simulink model "innoPWM_TestBench"  (R2022a)
settings: Solver=VariableStepAuto  StartTime=0.0  StopTime=0.5  FixedStep=1e-10  MaxStep=1e-4  RelTol=1e-3
PreLoadFcn:
  | clear;
  | dead_time= 5e-7;
  | T_sample = 1e-7;
  | fpwm= 8e3;
  | fel=200;
  | amplitude=0.1;
  | U_dc=800;
  | Iq_soll=200;
  | 
  | load('busdef.mat')
  | 
  | %**** Controller ****
  | L_filter = 70e-6;
  | R_losses = 1.74e-3;
  | PGain = L_filter*0.05*2*pi;
  | IGain = R_losses*0.05*2*pi;
  | 
  | %**** Deadtime Correction ****
  | Rds_on_module = 0.045/15;
  | 
  | %**** Filter ****
  | FilterQuality = 0.7071
InitFcn:
  | %%PGain = (L_filter*0.09*2*pi*f_pwm-R_losses)*0.45;
  | %%IGain = PGain*50/1.2; %% 25 = Period for ringing with too hight PGain
  | 
  | %%PGain = L_filter/(2*(1.5/fpwm));
  | %%IGain  = PGain*R_losses/L_filter;
undefined symbols (not defined in the file): DiscIntNeverNeededParam
libraries: nesl_utility x12, simulink x10, fl_lib x7, ee_lib x7, eeTransforms x2, spsFirstOrderFilterLib x1, spsRMSLib x1, simulink_extras x1, spspowerguiLib x1
settings Model: VariantFading=off  Creator=Z634594  LastModifiedBy=z634594
settings SolverCC: ZeroCrossAlgorithm=Adaptive  AlgebraicLoopSolver=TrustRegion
settings DataIOCC: ReturnWorkspaceOutputs=off
settings DebuggingCC: MergeDetectMultiDrivingBlocksExec=none  UnconnectedInputMsg=warning  UnconnectedOutputMsg=warning  UnconnectedLineMsg=warning  SFMachineParentedDataDiag=warning  ArithmeticOperatorsInVariantConditions=warning
settings SFSimCC: SimUseLocalCustomCode=off  CustomCodeUndefinedFunction=UseInterfaceOnly
settings RTWCC: RTWUseLocalCustomCode=off  DLArmComputeVersion=19.05
settings CodeAppCC: StateflowObjectComments=on

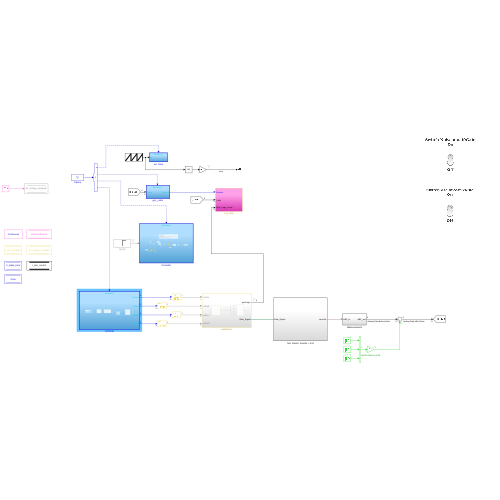
[thumbnail: Simulink's stored preview of the top-level diagram]
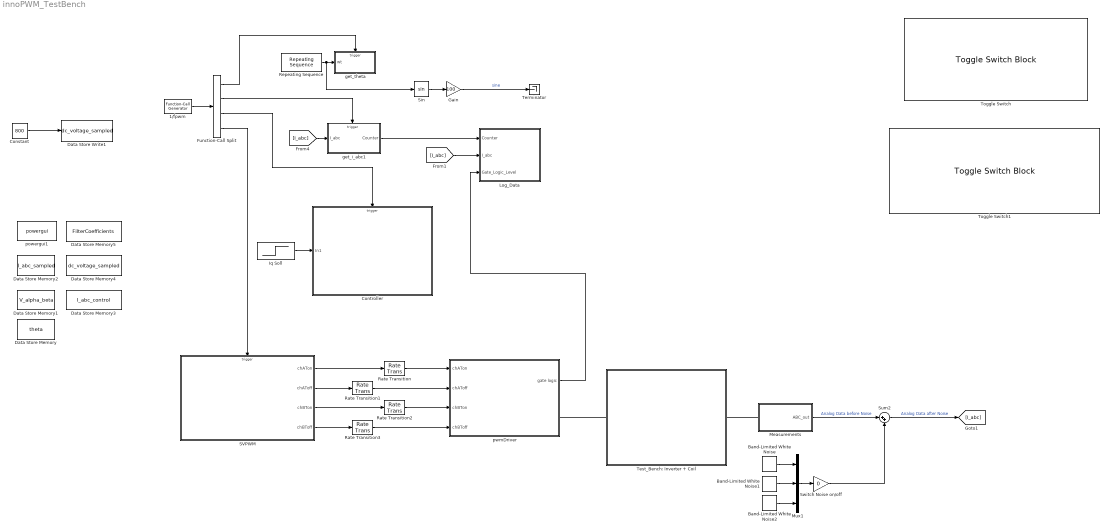
== system innoPWM_TestBench ==
  1/fpwm : simulink/Ports & Subsystems/Function-Call Generator  sample_time=1/fpwm  numberOfIterations=1  DisallowWideOutput=off
  Band-Limited White Noise : simulink/Sources/Band-Limited White Noise  Cov=[0.0004]  Ts=pi/2*1e-6  seed=[40000]
  Band-Limited White Noise1 : simulink/Sources/Band-Limited White Noise  Cov=[0.0004]  Ts=pi/2*1e-6  seed=[35000]
  Band-Limited White Noise2 : simulink/Sources/Band-Limited White Noise  Cov=[0.0004]  Ts=pi/2*1e-6  seed=[30000]
  Constant : Constant  Value=800
  Controller : Subsystem  TreatAsAtomicUnit=on
  Data Store Memory : DataStoreMemory  DataStoreName=theta  ReadBeforeWriteMsg=warning  WriteAfterWriteMsg=warning  WriteAfterReadMsg=warning  ShowAdditionalParam=off
  Data Store Memory1 : DataStoreMemory  DataStoreName=V_alpha_beta  ReadBeforeWriteMsg=warning  WriteAfterWriteMsg=warning  WriteAfterReadMsg=warning  InitialValue=[0 0]  ShowAdditionalParam=off
  Data Store Memory2 : DataStoreMemory  DataStoreName=I_abc_sampled  ReadBeforeWriteMsg=warning  WriteAfterWriteMsg=warning  WriteAfterReadMsg=warning  InitialValue=[0 0 0]  ShowAdditionalParam=off
  Data Store Memory3 : DataStoreMemory  DataStoreName=I_abc_control  ReadBeforeWriteMsg=warning  WriteAfterWriteMsg=warning  WriteAfterReadMsg=warning  InitialValue=[0 0 0]  ShowAdditionalParam=off
  Data Store Memory4 : DataStoreMemory  DataStoreName=dc_voltage_sampled  ReadBeforeWriteMsg=warning  WriteAfterWriteMsg=warning  WriteAfterReadMsg=warning  InitialValue=U_dc  ShowAdditionalParam=off
  Data Store Memory5 : DataStoreMemory  DataStoreName=FilterCoefficients  ReadBeforeWriteMsg=warning  WriteAfterWriteMsg=warning  WriteAfterReadMsg=warning  InitialValue=[1 0 0 0 0]  ShowAdditionalParam=off
  Data Store Write1 : DataStoreWrite  DataStoreName=dc_voltage_sampled  IndexOptions=Index vector (dialog)  Indices=1  OutputSizes=1
  Function-Call Split : FunctionCallSplit  IconShape=distinctive  NumOutputPorts=4  OutputPortLayout=default
  Gain : Gain  Gain=100
  Iq Soll : Step  Time=0.001  After=70  SampleTime=0
  Log_Data : Subsystem
  Measurements : Subsystem
  Mux1 : Mux  Inputs=3
  Rate Transition{,1..3} (4 alike) : RateTransition
  Repeating Sequence : simulink/Sources/Repeating Sequence  rep_seq_t=[0 1/fel]  rep_seq_y=[0 2*pi]
  SVPWM : Subsystem
  Sin : Trigonometry
  Sum2 : Sum  Inputs=|++
  Switch Noise on/off : Gain  Gain=0
  Terminator : Terminator
  Test_Bench: Inverter + Coil : Subsystem
  Toggle Switch : ToggleSwitchBlock
      settings: Values={{'Off', 'On'}, [0 1]}
  Toggle Switch1 : ToggleSwitchBlock
      settings: Values={{'Off', 'On'}, [0 1]}
  get_i_abc1 : Subsystem  TreatAsAtomicUnit=on
  get_theta : Subsystem  TreatAsAtomicUnit=on
  powergui1 : spspowerguiLib/powergui  Priority=1  SimulationMode=Continuous  SampleTime=1e-9  frequency=60  Iterations=50  frequencyindice=0  Pbase=100e6  ErrMax=1e-4  UnitsV=kV  UnitsW=MW  buscounter=0  FunctionMessages=off  echomessages=off  EnableUseOfTLC=off  CurrentSourceSwitches=off  DisableSnubberDevices=off  DisableRonSwitches=off  DisableVfSwitches=off  DisplayEquations=off  AutomaticDiscreteSolvers=off  SolverType=Tustin/Backward Euler (TBE)  Interpol=off  ExternalGateDelay=off  methode=off  Ts=100  x0status=blocks  SPID=on  SwTol=0  HookPort=off  NonlinearTolerance=1e-4  nMaxIteration=100  ContinueOnMaxIteration=off  RestoreLinks=warning  ResistiveCurrentMeasurement=off  Frange=[0:2:500]  Ylog=off  Xlog=on  ShowGrid=off  save=off  variable=ZData  structure=logsout  ZoomFFT=off  StartTime=0.01  cycles=10  DisplayStyle=1  fundamental=200  FreqAxis=off  MaxFrequency=10000  frequencyindicesteady=1  RmsSteady=1  display=off
  pwmDriver : Subsystem
  wires:
  Repeating Sequence/1 -> Sin/1, get_theta/1(wt)
  [I_abc] -> Log_Data/2(I_abc)
  Sum2/1 -> [I_abc]  "Analog Data after Noise"
  Band-Limited White Noise1/1 -> Mux1/2
  Band-Limited White Noise/1 -> Mux1/1
  Band-Limited White Noise2/1 -> Mux1/3
  Mux1/1 -> Switch Noise on/off/1
  Measurements/1(ABC_out) -> Sum2/1  "Analog Data before Noise"
  Switch Noise on/off/1 -> Sum2/2
  Constant/1 -> Data Store Write1/1
  get_i_abc1/1(Counter) -> Log_Data/1(Counter)
  pwmDriver/1(gate logic) -> Log_Data/3(Gate_Logic_Level)
  [I_abc] -> get_i_abc1/1(I_abc)
  1/fpwm/1 -> Function-Call Split/1
  Function-Call Split/1 -> get_theta/Trigger
  Function-Call Split/2 -> get_i_abc1/Trigger
  Function-Call Split/3 -> Controller/Trigger
  Function-Call Split/4 -> SVPWM/Trigger
  SVPWM/4(chBToff) -> Rate Transition3/1
  SVPWM/3(chBTon) -> Rate Transition2/1
  SVPWM/2(chAToff) -> Rate Transition1/1
  SVPWM/1(chATon) -> Rate Transition/1
  Rate Transition/1 -> pwmDriver/1(chATon)
  Rate Transition1/1 -> pwmDriver/2(chAToff)
  Rate Transition2/1 -> pwmDriver/3(chBTon)
  Rate Transition3/1 -> pwmDriver/4(chBToff)
  Sin/1 -> Gain/1
  Gain/1 -> Terminator/1  "sine"
  Iq Soll/1 -> Controller/1(In1)
  connections:
  Test_Bench: Inverter + Coil/LConn1 -- pwmDriver/RConn1
  Measurements/LConn1 -- Test_Bench: Inverter + Coil/RConn1

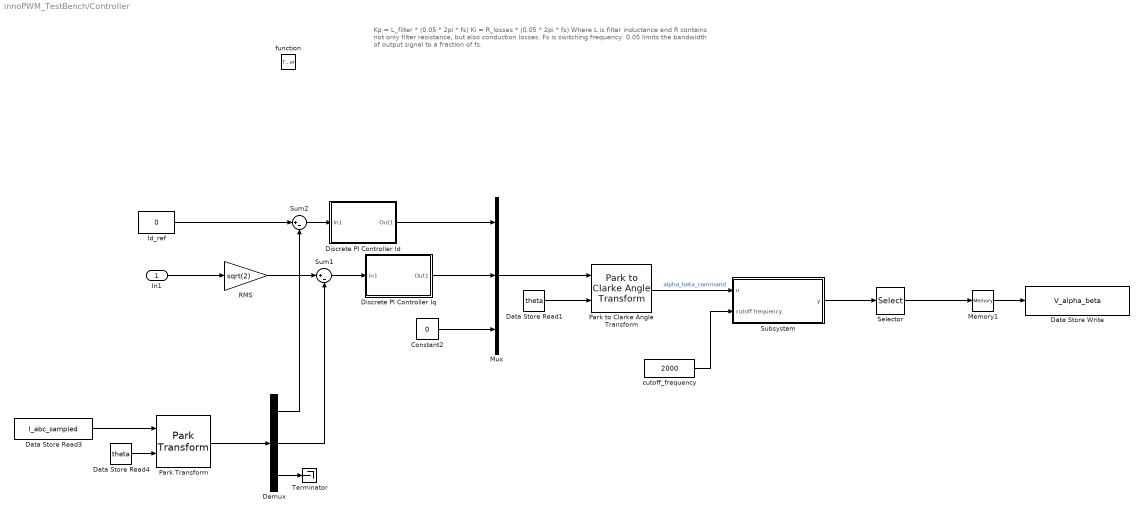
== system innoPWM_TestBench/Controller ==
  note: Kp = L_filter * (0.05 * 2pi * fs)
      |
      | Ki = R_losses * (0.05 * 2pi * fs)
      |
      | Where L is filter inductance and R contains not only filter resistance, but also conduction losses.
      | Fs is switching frequency.
      | 0.05 limits the bandwidth of output signal to a fraction of fs.
  In1 : Inport
  function : TriggerPort  TriggerType=function-call  VariantControl=Variant
  Constant2 : Constant  Value=0
  Data Store Read1 : DataStoreRead  DataStoreName=theta  IndexOptions=Index vector (dialog)  Indices=1  OutputSizes=1
  Data Store Read3 : DataStoreRead  DataStoreName=I_abc_sampled  IndexOptions=Index vector (dialog)  Indices=1  OutputSizes=1
  Data Store Read4 : DataStoreRead  DataStoreName=theta  IndexOptions=Index vector (dialog)  Indices=1  OutputSizes=1
  Data Store Write : DataStoreWrite  DataStoreName=V_alpha_beta  IndexOptions=Index vector (dialog)  Indices=1  OutputSizes=1
  Demux : Demux  Outputs=3
  Discrete PI Controller Id : Subsystem
  Discrete PI Controller Iq : Subsystem
  Id_ref : Constant  Value=0
  Memory1 : Memory  InheritSampleTime=on  LinearizeAsDelay=on
  Mux : Mux  Inputs=3
  Park Transform : eeTransforms/Park Transform  AxisAlignment=Q-axis  PowerInvariant=off
  Park to Clarke Angle Transform : eeTransforms/Park to Clarke Angle Transform  AxisAlignment=Q-axis
      settings: SourceProductBaseCode=PS
  RMS : Gain  Gain=sqrt(2)
  Selector : Selector  InputPortWidth=3  IndexOptions=Index vector (dialog)  Indices=[1 2]  OutputSizes=1
  Subsystem : Subsystem
  Sum1 : Sum  Inputs=|+-
  Sum2 : Sum  Inputs=|+-
  Terminator : Terminator
  cutoff_frequency : Constant  Value=2000
  wires:
  Demux/1 -> Sum2/2
  Mux/1 -> Park to Clarke Angle Transform/1
  Demux/3 -> Terminator/1
  Demux/2 -> Sum1/2
  Constant2/1 -> Mux/3
  Sum2/1 -> Discrete PI Controller Id/1(In1)
  Sum1/1 -> Discrete PI Controller Iq/1(In1)
  Discrete PI Controller Iq/1(Out1) -> Mux/2
  Data Store Read3/1 -> Park Transform/1
  Data Store Read4/1 -> Park Transform/2
  Data Store Read1/1 -> Park to Clarke Angle Transform/2
  Memory1/1 -> Data Store Write/1
  Discrete PI Controller Id/1(Out1) -> Mux/1
  Park Transform/1 -> Demux/1
  Selector/1 -> Memory1/1
  Id_ref/1 -> Sum2/1
  In1/1 -> RMS/1
  RMS/1 -> Sum1/1
  cutoff_frequency/1 -> Subsystem/2(cutoff frequency)
  Park to Clarke Angle Transform/1 -> Subsystem/1(u)  "alpha_beta_command"
  Subsystem/1(y) -> Selector/1

== system innoPWM_TestBench/Log_Data ==
  Counter : Inport
  I_abc : Inport  Port=2
  Gate_Logic_Level : Inport  Port=3
  Data Store Read1 : DataStoreRead  DataStoreName=I_abc_sampled  IndexOptions=Index vector (dialog)  Indices=1  OutputSizes=1
  Data Store Read2 : DataStoreRead  DataStoreName=I_abc_control  IndexOptions=Index vector (dialog)  Indices=1  OutputSizes=1
  Delay : Delay  DelayLength=1  SampleTime=T_sample
  Gain : Gain  Gain=50
  Logical Operator : Logic  Operator=XOR  AllPortsSameDT=off  OutDataTypeStr=boolean
  Product : Product
  Scope1 : Scope  NumInputPorts=3
  Scope6 : Scope  NumInputPorts=5
  wires:
  Delay/1 -> Scope1/2, Logical Operator/1
  Data Store Read1/1 -> Product/2, Scope6/1
  Counter/1 -> Scope1/1, Logical Operator/2, Delay/1
  Product/1 -> Scope6/3
  Logical Operator/1 -> Scope1/3, Product/1
  Gain/1 -> Scope6/4
  I_abc/1 -> Scope6/2
  Gate_Logic_Level/1 -> Gain/1
  Data Store Read2/1 -> Scope6/5

== system innoPWM_TestBench/Measurements ==
  First-Order Filter : spsFirstOrderFilterLib/First-Order Filter  FilterType=Lowpass  Tc=25e-6  Ts=0  Initialize=off  Vac_Init=[0, 0, 60]  Vdc_Init=0  PlotResponse=off  FreqRange="[0,  200,  1]"
  PS-Simulink Converter1 : nesl_utility/PS-Simulink Converter  PhysicalDomain=network_engine_domain  SubClassName=ps_output  LeftPortType=input  RightPortType=output  PseudoPeriodic=off  Frequencies=[]  VectorFormat=1-D array  Unit=1  AffineConversion=off
      settings: SourceProductBaseCode=SS,PW,VE
  RMS : spsRMSLib/RMS  TrueRMS=on  Freq=fel  RMSInit=0  Ts=0
  Terminator : Terminator
  Terminator1 : Terminator
  ABC_in : PMIOPort  Side=Left
  ABC_out : Outport  VectorParamsAs1DForOutWhenUnconnected=off
  wires:
  PS-Simulink Converter1/1 -> RMS/1, First-Order Filter/1, ABC_out/1
  RMS/1 -> Terminator/1  "rmsCurrent3Phase"
  First-Order Filter/1 -> Terminator1/1  "phaseCurrent3Phase"
  connections:
  PS-Simulink Converter1/LConn1 -- ABC_in/RConn1

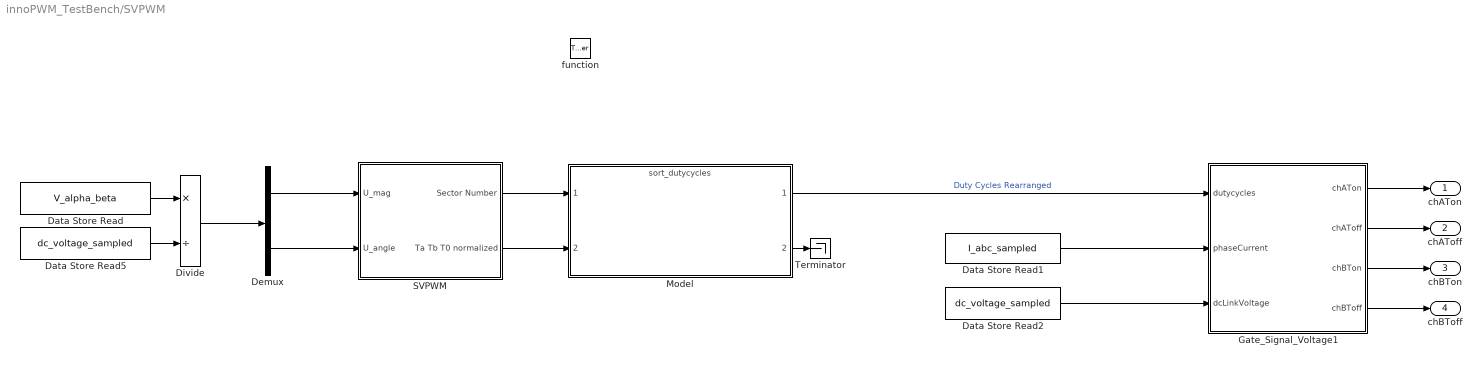
== system innoPWM_TestBench/SVPWM ==
  function : TriggerPort  TriggerType=function-call  VariantControl=(inherit)
  Data Store Read : DataStoreRead  DataStoreName=V_alpha_beta  IndexOptions=Index vector (dialog)  Indices=1  OutputSizes=1
  Data Store Read1 : DataStoreRead  DataStoreName=I_abc_sampled  IndexOptions=Index vector (dialog)  Indices=1  OutputSizes=1
  Data Store Read2 : DataStoreRead  DataStoreName=dc_voltage_sampled  IndexOptions=Index vector (dialog)  Indices=1  OutputSizes=1
  Data Store Read5 : DataStoreRead  DataStoreName=dc_voltage_sampled  IndexOptions=Index vector (dialog)  Indices=1  OutputSizes=1
  Demux : Demux  Outputs=2
  Divide : Product  Inputs=*/
  Gate_Signal_Voltage1 : Subsystem
  Model : ModelReference  ModelNameDialog=sort_dutycycles.slx  SimulationMode=Normal  ModelReferenceVersion=1.5
  SVPWM : Subsystem
  Terminator : Terminator
  chATon : Outport
  chAToff : Outport  Port=2
  chBTon : Outport  Port=3
  chBToff : Outport  Port=4
  wires:
  Divide/1 -> Demux/1
  Data Store Read5/1 -> Divide/2
  SVPWM/1(Sector Number) -> Model/1
  SVPWM/2(Ta Tb T0 normalized) -> Model/2
  Data Store Read/1 -> Divide/1
  Demux/2 -> SVPWM/2(U_angle)
  Model/2 -> Terminator/1
  Demux/1 -> SVPWM/1(U_mag)
  Model/1 -> Gate_Signal_Voltage1/1(dutycycles)  "Duty Cycles Rearranged"
  Data Store Read1/1 -> Gate_Signal_Voltage1/2(phaseCurrent)
  Data Store Read2/1 -> Gate_Signal_Voltage1/3(dcLinkVoltage)
  Gate_Signal_Voltage1/1(chATon) -> chATon/1
  Gate_Signal_Voltage1/2(chAToff) -> chAToff/1
  Gate_Signal_Voltage1/3(chBTon) -> chBTon/1
  Gate_Signal_Voltage1/4(chBToff) -> chBToff/1

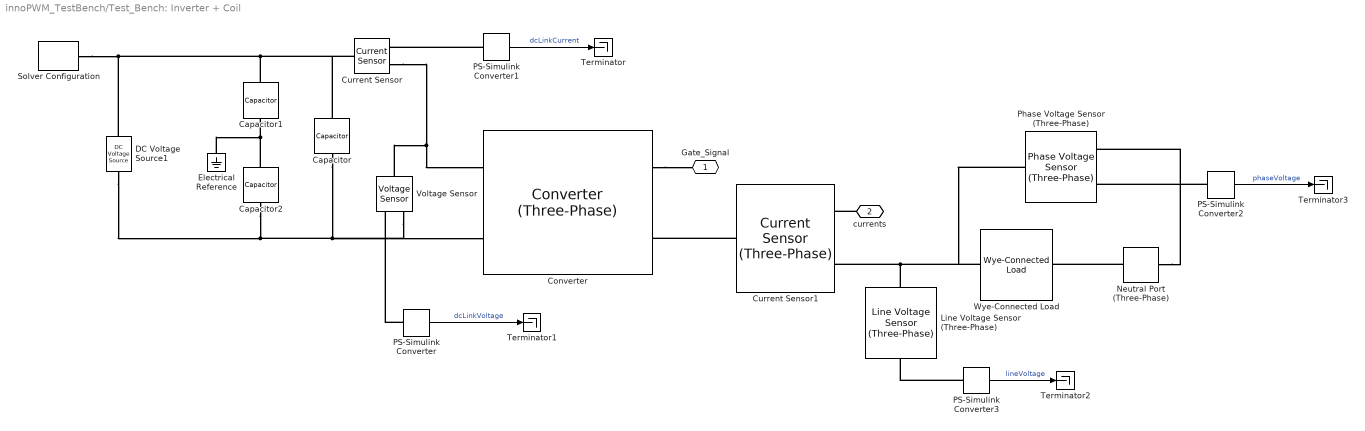
== system innoPWM_TestBench/Test_Bench: Inverter + Coil ==
  Capacitor : fl_lib/Electrical/Electrical Elements/Capacitor  c=550e-6 F  r=1e-6 Ohm  g=0 1/Ohm  i_specify=off  i_priority=None  i=0 A  i_nominal_specify=off  i_nominal_unit=A  i_nominal_value=1  v_specify=off  v_priority=None  v=0 V  v_nominal_specify=off  v_nominal_unit=V  v_nominal_value=1  vc_specify=on  vc_priority=High  vc=U_dc V  vc_nominal_specify=off  vc_nominal_unit=V  vc_nominal_value=1
      settings: SourceProductBaseCode=PW,SS,VE
  Capacitor1 : fl_lib/Electrical/Electrical Elements/Capacitor  c=100e-9 F  r=1e-6 Ohm  g=0 1/Ohm  i_specify=off  i_priority=None  i=0 A  i_nominal_specify=off  i_nominal_unit=A  i_nominal_value=1  v_specify=off  v_priority=None  v=0 V  v_nominal_specify=off  v_nominal_unit=V  v_nominal_value=1  vc_specify=on  vc_priority=High  vc=U_dc/2 V  vc_nominal_specify=off  vc_nominal_unit=V  vc_nominal_value=1
      settings: SourceProductBaseCode=PW,SS,VE
  Capacitor2 : fl_lib/Electrical/Electrical Elements/Capacitor  c=100e-9 F  r=1e-6 Ohm  g=0 1/Ohm  i_specify=off  i_priority=None  i=0 A  i_nominal_specify=off  i_nominal_unit=A  i_nominal_value=1  v_specify=off  v_priority=None  v=0 V  v_nominal_specify=off  v_nominal_unit=V  v_nominal_value=1  vc_specify=on  vc_priority=High  vc=U_dc/2 V  vc_nominal_specify=off  vc_nominal_unit=V  vc_nominal_value=1
      settings: SourceProductBaseCode=PW,SS,VE
  Converter : ee_lib/Semiconductors & Converters/Converters/Converter (Three-Phase)  port_option=ee.enum.threePhasePort.composite  device_type=ee.enum.converters.switchingdevice.mosfet  Vf=0.8 V  Ron=0.001 Ohm  Rds=Rds_on_module Ohm  Goff=1e-9 1/Ohm  Vgt=1 V  Vgt_off=-1 V  Ih=1 A  Vth=4 V  diode_param=ee.enum.converters.protectiondiode.nodynamics  diode_Vf=2 V  diode_Ron=Rds_on_module Ohm  diode_Goff=1e-9 1/Ohm  diode_C=50 nF  diode_iRM=-235 A  diode_iF=300 A  diode_idot=-50 A/us  diode_trr_param=ee.enum.converters.diodetrr.trr_factor  diode_trr_factor=3  diode_trr=15 us  diode_Qrr=1.5e+3 s*uA  snubber_type=ee.enum.converters.snubber.exclude  Cs=1e-6 F  Rs=0.01 Ohm
      settings: SourceProductBaseCode=PS
  Current Sensor : fl_lib/Electrical/Electrical Sensors/Current Sensor
      settings: SourceProductBaseCode=PW,SS,VE
  Current Sensor1 : ee_lib/Sensors & Transducers/Current Sensor (Three-Phase)
  DC Voltage Source1 : fl_lib/Electrical/Electrical Sources/DC Voltage Source  v0=U_dc V
      settings: SourceProductBaseCode=PW,SS,VE
  Electrical Reference : fl_lib/Electrical/Electrical Elements/Electrical Reference
      settings: SourceProductBaseCode=PW,SS,VE
  Line Voltage Sensor (Three-Phase) : ee_lib/Sensors & Transducers/Line Voltage Sensor (Three-Phase)
      settings: SourceProductBaseCode=PS
  Neutral Port (Three-Phase) : ee_lib/Connectors & References/Neutral Port (Three-Phase)  G_parasitic=1e-12 1/Ohm
      settings: SourceProductBaseCode=PS  InternalSimscapePortConfiguration="{\"Bottom\":[],\"Left\":[{\"id\":\"N\",\"label\":\"~\",\"type\":\"foundation.electrical.three_phase\"}],\"Right\":[{\"id\":\"n\",\"label\":\"n\",\"type\":\"foundation.electrical.electrical\"}],\"Top\":[]}"
  PS-Simulink Converter{,1..3} (4 alike) : nesl_utility/PS-Simulink Converter  PhysicalDomain=network_engine_domain  SubClassName=ps_output  LeftPortType=input  RightPortType=output  PseudoPeriodic=off  Frequencies=[]  VectorFormat=1-D array  Unit=1  AffineConversion=off
      settings: SourceProductBaseCode=SS,PW,VE
  Phase Voltage Sensor (Three-Phase) : ee_lib/Sensors & Transducers/Phase Voltage Sensor (Three-Phase)
      settings: SourceProductBaseCode=PS
  Solver Configuration : nesl_utility/Solver Configuration  PhysicalDomain=network_engine_domain  SubClassName=solver  LeftPortType=input  RightPortType=generic  Tones=[]  Harmonics=[]  SimulateNoise=off  Profile=off  UseLocalSampling=off  EnableSwitchedLinearOptims=on  FrequencyDomain=off  UseCCode=off  RelTol=0.001  AbsTol=1e-06  MinStep=1e-09  ToWorkspace=off  RevertToSquareIcSolve=off  NumHomotopyIterations=100  PhasorMode=off  PhasorModeNumHarmonics=1  IndexReductionMethod=DerivativeReplacement  DoDC=off  ResidualTolerance=1e-09  UseLocalSolver=off  LocalSolverChoice=NE_BACKWARD_EULER_ADVANCER  LocalSolverSampleTime=0.001  DoFixedCost=off  MaxNonlinIter=3  MaxModeIter=2  ComputeImpulses=off  ImpulseIterations=2  LinearAlgebra=Sparse  LinearAlgebraNumThread=0  EquationFormulation=NE_TIME_EF  DelaysMemoryBudget=1024  AutomaticFiltering=on  FilteringTimeConstant=0.001  PartitionStorageMethod=AS_NEEDED  PartitionMemoryBudget=1024  PartitionMethod=FAST
      settings: SourceProductBaseCode=SS,PW,VE
  Terminator{,1..3} (4 alike) : Terminator
  Voltage Sensor : fl_lib/Electrical/Electrical Sensors/Voltage Sensor
      settings: SourceProductBaseCode=PW,SS,VE
  Wye-Connected Load : ee_lib/Passive/RLC Assemblies/Wye-Connected Load  parameterization=ee.enum.rlc.parameterization.direct  component_structure=ee.enum.rlc.structure.SeriesRL  component_structure_PQ=ee.enum.rlc.structure.SeriesRL  R=1.74e-3 Ohm  L=70e-6 H  C=1e-6 F  VRated=24e3 V  FRated=60 Hz  P=1e3 W  Qpos=1e2 V*A  Qneg=-1e2 V*A  R_parasitic=1e-6 Ohm  G_parasitic=1e-9 1/Ohm  R_parasitic_PQ=1e-6 Ohm  G_parasitic_PQ=1e-6 1/Ohm  Vmag0=24e3 V  Vang0=0 deg  Freq0=60 Hz  IL_specify=off  IL_priority=High  IL=[ 0 0 0 ] A  IL_nominal_specify=off  IL_nominal_unit=A  IL_nominal_value=1  VC_specify=off  VC_priority=High  VC=[ 0 0 0 ] V  VC_nominal_specify=off  VC_nominal_unit=V  VC_nominal_value=1
      settings: SourceProductBaseCode=PS
  Gate_Signal : PMIOPort  Side=Left
  currents : PMIOPort  Port=2  Side=Right
  wires:
  PS-Simulink Converter1/1 -> Terminator/1  "dcLinkCurrent"
  PS-Simulink Converter/1 -> Terminator1/1  "dcLinkVoltage"
  PS-Simulink Converter3/1 -> Terminator2/1  "lineVoltage"
  PS-Simulink Converter2/1 -> Terminator3/1  "phaseVoltage"
  connections:
  Current Sensor1/LConn1 -- Converter/LConn2
  Converter/LConn1 -- Gate_Signal/RConn1
  Capacitor/RConn1 -- Converter/RConn2 -- Voltage Sensor/RConn2 -- DC Voltage Source1/RConn1 -- Capacitor2/RConn1
  Current Sensor/RConn2 -- Converter/RConn1 -- Voltage Sensor/LConn1
  PS-Simulink Converter/LConn1 -- Voltage Sensor/RConn1
  PS-Simulink Converter1/LConn1 -- Current Sensor/RConn1
  Capacitor1/LConn1 -- Capacitor/LConn1 -- Current Sensor/LConn1 -- DC Voltage Source1/LConn1 -- Solver Configuration/RConn1
  currents/RConn1 -- Current Sensor1/RConn1
  PS-Simulink Converter2/LConn1 -- Phase Voltage Sensor (Three-Phase)/RConn1
  Capacitor2/LConn1 -- Electrical Reference/LConn1 -- Capacitor1/RConn1
  PS-Simulink Converter3/LConn1 -- Line Voltage Sensor (Three-Phase)/RConn1
  Line Voltage Sensor (Three-Phase)/LConn1 -- Wye-Connected Load/LConn1 -- Phase Voltage Sensor (Three-Phase)/LConn1 -- Current Sensor1/RConn2
  Neutral Port (Three-Phase)/LConn1 -- Phase Voltage Sensor (Three-Phase)/RConn2
  Neutral Port (Three-Phase)/RConn1 -- Wye-Connected Load/RConn1

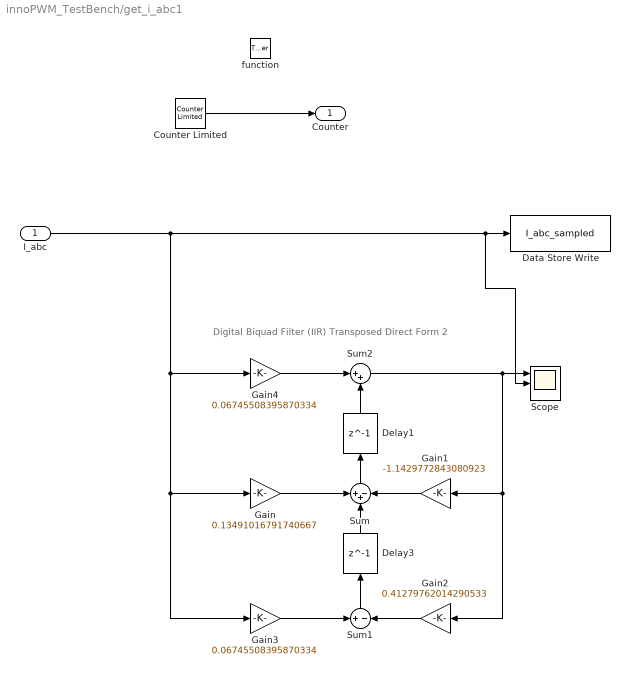
== system innoPWM_TestBench/get_i_abc1 ==
  note: Digital Biquad Filter (IIR)
      | Transposed Direct Form 2
  I_abc : Inport
  function : TriggerPort  TriggerType=function-call  VariantControl=Variant
  Counter Limited : simulink/Sources/Counter Limited  uplimit=1  tsamp=-1
  Data Store Write : DataStoreWrite  DataStoreName=I_abc_sampled  IndexOptions=Index vector (dialog)  Indices=1  OutputSizes=1
  Delay1 : Delay  DelayLength=1
  Delay3 : Delay  DelayLength=1
  Gain : Gain  Gain=0.13491016791740667
  Gain1 : Gain  Gain=-1.1429772843080923
  Gain2 : Gain  Gain=0.41279762014290533
  Gain3 : Gain  Gain=0.06745508395870334
  Gain4 : Gain  Gain=0.06745508395870334
  Scope : Scope  NumInputPorts=3
  Sum : Sum  Inputs=++-
  Sum1 : Sum  Inputs=+|-
  Sum2 : Sum  Inputs=|++
  Counter : Outport  VectorParamsAs1DForOutWhenUnconnected=off
  wires:
  Counter Limited/1 -> Counter/1
  Gain/1 -> Sum/1
  Gain1/1 -> Sum/3
  Gain3/1 -> Sum1/1
  Gain2/1 -> Sum1/2
  Gain4/1 -> Sum2/1
  Delay1/1 -> Sum2/2
  Sum/1 -> Delay1/1
  Delay3/1 -> Sum/2
  Sum1/1 -> Delay3/1
  Sum2/1 -> Gain2/1, Gain1/1, Scope/1
  I_abc/1 -> Scope/2, Data Store Write/1, Gain4/1, Gain/1, Gain3/1

== system innoPWM_TestBench/get_theta ==
  wt : Inport
  function : TriggerPort  TriggerType=function-call  VariantControl=Variant
  Data Store Write : DataStoreWrite  DataStoreName=theta  IndexOptions=Index vector (dialog)  Indices=1  OutputSizes=1
  wires:
  wt/1 -> Data Store Write/1

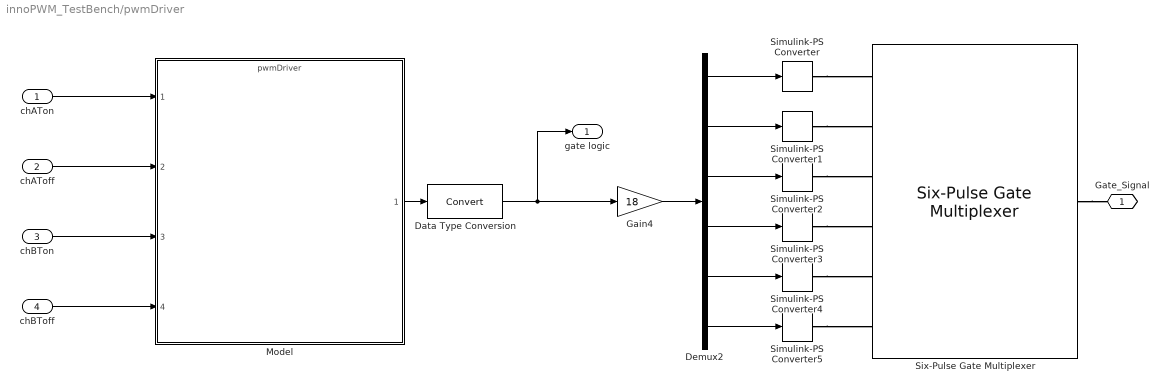
== system innoPWM_TestBench/pwmDriver ==
  chATon : Inport
  chAToff : Inport  Port=2
  chBTon : Inport  Port=3
  chBToff : Inport  Port=4
  Data Type Conversion : DataTypeConversion  SaturateOnIntegerOverflow=off  RndMeth=Floor
  Demux2 : Demux  Outputs=6
  Gain4 : Gain  Gain=18
  Model : ModelReference  ModelNameDialog=pwmDriver.slx  SimulationMode=Normal  ModelReferenceVersion=1.3
  Simulink-PS Converter{,1..5} (6 alike) : nesl_utility/Simulink-PS Converter  PhysicalDomain=network_engine_domain  SubClassName=ps_input  LeftPortType=input  RightPortType=output  PseudoPeriodic=off  Frequencies=[]  NoiseDistribution=none  NoiseParameters=[]  Unit=1  AffineConversion=off  FilteringAndDerivatives=provide  SimscapeFilterOrder=1  InputFilterTimeConstant=0.001  UdotUserProvided=0
      settings: SourceProductBaseCode=SS,PW,VE
  Six-Pulse Gate Multiplexer : ee_lib/Semiconductors & Converters/Converters/Six-Pulse Gate Multiplexer  port_option=ee.enum.controlport.ps
      settings: SourceProductBaseCode=PS
  Gate_Signal : PMIOPort  Side=Right
  gate logic : Outport  VectorParamsAs1DForOutWhenUnconnected=off
  wires:
  chBToff/1 -> Model/4
  Data Type Conversion/1 -> gate logic/1, Gain4/1
  chAToff/1 -> Model/2
  Model/1 -> Data Type Conversion/1
  chBTon/1 -> Model/3
  Gain4/1 -> Demux2/1
  chATon/1 -> Model/1
  Demux2/1 -> Simulink-PS Converter/1
  Demux2/2 -> Simulink-PS Converter1/1
  Demux2/3 -> Simulink-PS Converter2/1
  Demux2/4 -> Simulink-PS Converter3/1
  Demux2/5 -> Simulink-PS Converter4/1
  Demux2/6 -> Simulink-PS Converter5/1
  connections:
  Simulink-PS Converter1/RConn1 -- Six-Pulse Gate Multiplexer/LConn2
  Simulink-PS Converter5/RConn1 -- Six-Pulse Gate Multiplexer/LConn6
  Simulink-PS Converter2/RConn1 -- Six-Pulse Gate Multiplexer/LConn3
  Six-Pulse Gate Multiplexer/RConn1 -- Gate_Signal/RConn1
  Simulink-PS Converter4/RConn1 -- Six-Pulse Gate Multiplexer/LConn5
  Simulink-PS Converter/RConn1 -- Six-Pulse Gate Multiplexer/LConn1
  Simulink-PS Converter3/RConn1 -- Six-Pulse Gate Multiplexer/LConn4

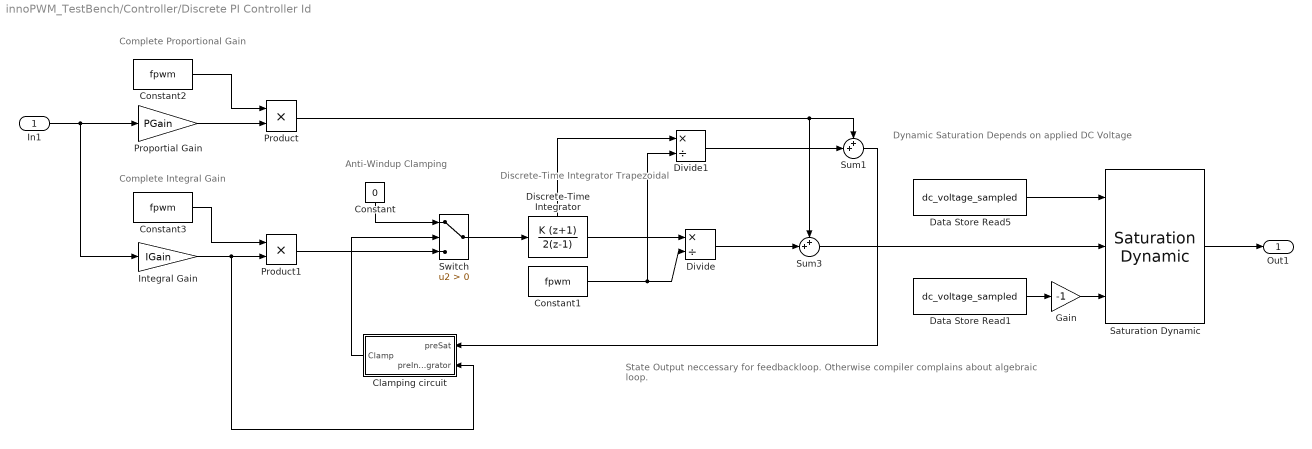
== system innoPWM_TestBench/Controller/Discrete PI Controller Id ==
  note: State Output neccessary for feedbackloop. Otherwise compiler complains about algebraic loop.
  note: Complete Proportional Gain
  note: Discrete-Time Integrator Trapezoidal
  note: Complete Integral Gain
  note: Anti-Windup Clamping
  note: Dynamic Saturation
      | Depends on applied DC Voltage
  In1 : Inport
  Clamping circuit : Subsystem
  Constant : Constant  DisableCoverage=on  Value=0  OutDataTypeStr=Inherit: Inherit via back propagation  PreserveConstantTs=on
  Constant1 : Constant  Value=fpwm
  Constant2 : Constant  Value=fpwm
  Constant3 : Constant  Value=fpwm
  Data Store Read1 : DataStoreRead  DataStoreName=dc_voltage_sampled  IndexOptions=Index vector (dialog)  Indices=1  OutputSizes=1
  Data Store Read5 : DataStoreRead  DataStoreName=dc_voltage_sampled  IndexOptions=Index vector (dialog)  Indices=1  OutputSizes=1
  Discrete-Time Integrator : DiscreteIntegrator  IntegratorMethod=Accumulation: Trapezoidal  SampleTime=-1  ShowStatePort=on  ICPrevOutput=DiscIntNeverNeededParam  ICPrevScaledInput=DiscIntNeverNeededParam
  Divide : Product  Inputs=*/
  Divide1 : Product  Inputs=*/
  Gain : Gain  Gain=-1
  Integral Gain : Gain  Gain=IGain
  Product : Product
  Product1 : Product
  Proportial Gain : Gain  Gain=PGain
  Saturation Dynamic : simulink/Discontinuities/Saturation Dynamic  OutMin=[]  OutMax=[]  OutDataTypeStr=Inherit: Same as second input  OutDataType=fixdt(1, 16)  OutScaling=2^-10  DoSatur=off
  Sum1 : Sum  Inputs=++|
  Sum3 : Sum  Inputs=++|
  Switch : Switch  Criteria=u2 > Threshold  SaturateOnIntegerOverflow=off
  Out1 : Outport  VectorParamsAs1DForOutWhenUnconnected=off
  wires:
  Constant/1 -> Switch/1
  Clamping circuit/1(Clamp) -> Switch/2
  In1/1 -> Proportial Gain/1, Integral Gain/1
  Discrete-Time Integrator/1 -> Divide/1
  Switch/1 -> Discrete-Time Integrator/1
  Constant1/1 -> Divide/2, Divide1/2
  Sum1/1 -> Clamping circuit/1(preSat)
  Data Store Read5/1 -> Saturation Dynamic/1
  Data Store Read1/1 -> Gain/1
  Gain/1 -> Saturation Dynamic/3
  Saturation Dynamic/1 -> Out1/1
  Sum3/1 -> Saturation Dynamic/2
  Proportial Gain/1 -> Product/2
  Constant2/1 -> Product/1
  Integral Gain/1 -> Clamping circuit/2(preIntegrator), Product1/2
  Constant3/1 -> Product1/1
  Divide/1 -> Sum3/2
  Divide1/1 -> Sum1/2
  Discrete-Time Integrator/State -> Divide1/1
  Product/1 -> Sum3/1, Sum1/1
  Product1/1 -> Switch/3

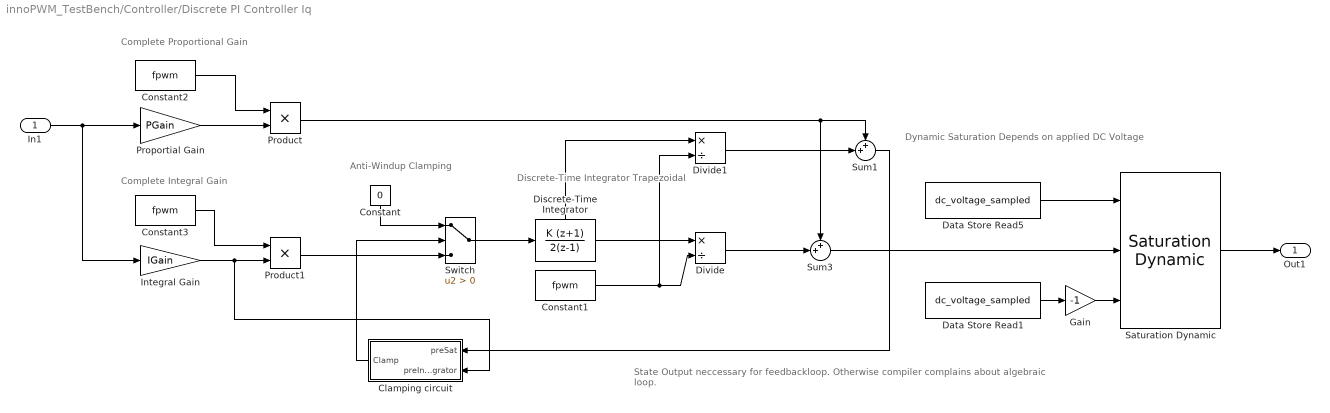
== system innoPWM_TestBench/Controller/Discrete PI Controller Iq ==
  note: Dynamic Saturation
      | Depends on applied DC Voltage
  note: Anti-Windup Clamping
  note: Complete Integral Gain
  note: Discrete-Time Integrator Trapezoidal
  note: Complete Proportional Gain
  note: State Output neccessary for feedbackloop. Otherwise compiler complains about algebraic loop.
  In1 : Inport
  Clamping circuit : Subsystem
  Constant : Constant  DisableCoverage=on  Value=0  OutDataTypeStr=Inherit: Inherit via back propagation  PreserveConstantTs=on
  Constant1 : Constant  Value=fpwm
  Constant2 : Constant  Value=fpwm
  Constant3 : Constant  Value=fpwm
  Data Store Read1 : DataStoreRead  DataStoreName=dc_voltage_sampled  IndexOptions=Index vector (dialog)  Indices=1  OutputSizes=1
  Data Store Read5 : DataStoreRead  DataStoreName=dc_voltage_sampled  IndexOptions=Index vector (dialog)  Indices=1  OutputSizes=1
  Discrete-Time Integrator : DiscreteIntegrator  IntegratorMethod=Accumulation: Trapezoidal  SampleTime=-1  ShowStatePort=on  ICPrevOutput=DiscIntNeverNeededParam  ICPrevScaledInput=DiscIntNeverNeededParam
  Divide : Product  Inputs=*/
  Divide1 : Product  Inputs=*/
  Gain : Gain  Gain=-1
  Integral Gain : Gain  Gain=IGain
  Product : Product
  Product1 : Product
  Proportial Gain : Gain  Gain=PGain
  Saturation Dynamic : simulink/Discontinuities/Saturation Dynamic  OutMin=[]  OutMax=[]  OutDataTypeStr=Inherit: Same as second input  OutDataType=fixdt(1, 16)  OutScaling=2^-10  DoSatur=off
  Sum1 : Sum  Inputs=++|
  Sum3 : Sum  Inputs=++|
  Switch : Switch  Criteria=u2 > Threshold  SaturateOnIntegerOverflow=off
  Out1 : Outport  VectorParamsAs1DForOutWhenUnconnected=off
  wires:
  Constant3/1 -> Product1/1
  Integral Gain/1 -> Clamping circuit/2(preIntegrator), Product1/2
  Constant2/1 -> Product/1
  Proportial Gain/1 -> Product/2
  Saturation Dynamic/1 -> Out1/1
  Gain/1 -> Saturation Dynamic/3
  Data Store Read1/1 -> Gain/1
  Data Store Read5/1 -> Saturation Dynamic/1
  Sum1/1 -> Clamping circuit/1(preSat)
  Constant1/1 -> Divide1/2, Divide/2
  Switch/1 -> Discrete-Time Integrator/1
  Discrete-Time Integrator/1 -> Divide/1
  In1/1 -> Integral Gain/1, Proportial Gain/1
  Clamping circuit/1(Clamp) -> Switch/2
  Constant/1 -> Switch/1
  Divide/1 -> Sum3/2
  Discrete-Time Integrator/State -> Divide1/1
  Divide1/1 -> Sum1/2
  Sum3/1 -> Saturation Dynamic/2
  Product/1 -> Sum3/1, Sum1/1
  Product1/1 -> Switch/3

== system innoPWM_TestBench/Controller/Subsystem ==
  u : Inport
  cutoff frequency : Inport  Port=2
  Constant : Constant  Value=fpwm
  MATLAB Function1 : MATLAB Function  TreatAsAtomicUnit=on
  MATLAB Function2 : MATLAB Function  TreatAsAtomicUnit=on
  Product1 : Product
  Product4 : Product
  Sum : Sum  Inputs=|++
  Sum3 : Sum  Inputs=+|+
  Unit Delay : UnitDelay  SampleTime=-1  HasFrameUpgradeWarning=on
  y : Outport  VectorParamsAs1DForOutWhenUnconnected=off
  wires:
  u/1 -> Sum/1, Sum3/1
  Sum/1 -> Product1/2, Product4/2
  Product4/1 -> Sum3/2
  Sum3/1 -> Unit Delay/1
  cutoff frequency/1 -> MATLAB Function2/1(w), MATLAB Function1/1(fc)
  Unit Delay/1 -> Sum/2
  MATLAB Function2/2(a) -> Product4/1
  MATLAB Function2/1(g) -> Product1/1
  Product1/1 -> y/1
  MATLAB Function1/1(tau) -> MATLAB Function2/2(tau)
  Constant/1 -> MATLAB Function1/2(fpwm)

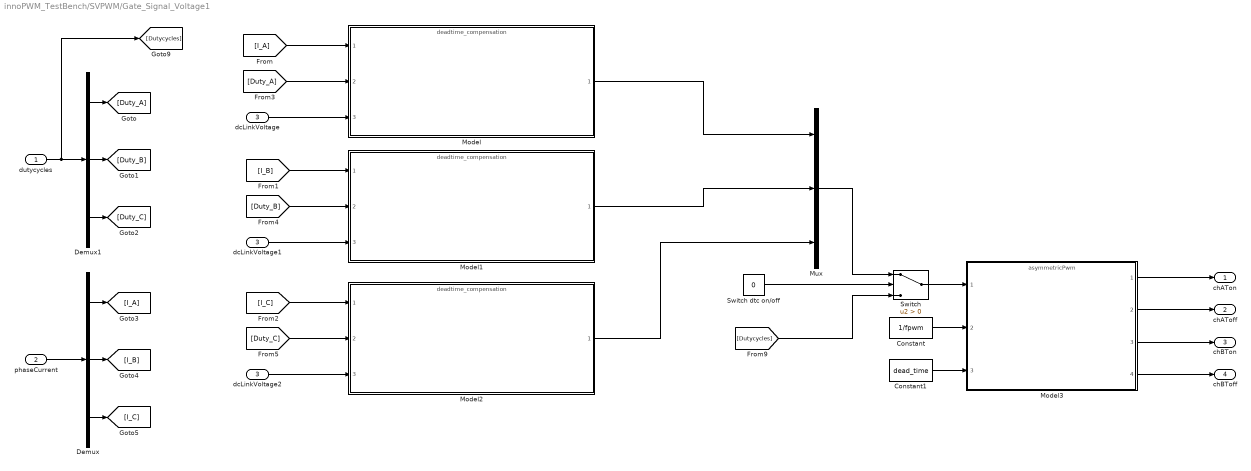
== system innoPWM_TestBench/SVPWM/Gate_Signal_Voltage1 ==
  dutycycles : Inport
  phaseCurrent : Inport  Port=2
  dcLinkVoltage : Inport  Port=3
  Constant : Constant  Value=1/fpwm
  Constant1 : Constant  Value=dead_time
  Demux : Demux  Outputs=3
  Demux1 : Demux  Outputs=3
  Model : ModelReference  ModelNameDialog=deadtime_compensation.slx  SimulationMode=Normal  ModelReferenceVersion=8.4
  Model1 : ModelReference  ModelNameDialog=deadtime_compensation.slx  SimulationMode=Normal  ModelReferenceVersion=8.4
  Model2 : ModelReference  ModelNameDialog=deadtime_compensation.slx  SimulationMode=Normal  ModelReferenceVersion=8.4
  Model3 : ModelReference  ModelNameDialog=asymmetricPwm.slx  SimulationMode=Normal  ModelReferenceVersion=1.3
  Mux : Mux  Inputs=3
  Switch : Switch  Criteria=u2 > Threshold  SaturateOnIntegerOverflow=off  InputSameDT=off
  Switch dtc on/off : Constant  Value=0
  dcLinkVoltage1 : InportShadow  Port=3
  dcLinkVoltage2 : InportShadow  Port=3
  chATon : Outport
  chAToff : Outport  Port=2
  chBTon : Outport  Port=3
  chBToff : Outport  Port=4
  wires:
  phaseCurrent/1 -> Demux/1
  Demux1/1 -> [Duty_A]
  Demux1/2 -> [Duty_B]
  Demux1/3 -> [Duty_C]
  Demux/1 -> [I_A]
  Demux/2 -> [I_B]
  Demux/3 -> [I_C]
  [I_A] -> Model/1
  [Duty_A] -> Model/2
  Model/1 -> Mux/1
  [I_B] -> Model1/1
  [Duty_B] -> Model1/2
  Model1/1 -> Mux/2
  [Duty_C] -> Model2/2
  Switch dtc on/off/1 -> Switch/2
  [Dutycycles] -> Switch/3
  Mux/1 -> Switch/1
  dutycycles/1 -> Demux1/1, [Dutycycles]
  Model2/1 -> Mux/3
  Switch/1 -> Model3/1
  Model3/2 -> chAToff/1
  Model3/4 -> chBToff/1
  Model3/3 -> chBTon/1
  [I_C] -> Model2/1
  dcLinkVoltage1/1 -> Model1/3
  dcLinkVoltage/1 -> Model/3
  dcLinkVoltage2/1 -> Model2/3
  Constant/1 -> Model3/2
  Constant1/1 -> Model3/3
  Model3/1 -> chATon/1

== system innoPWM_TestBench/SVPWM/SVPWM ==
  U_mag : Inport
  U_angle : Inport  Port=2
  Constant4 : Constant  Value=fel
  Constant5 : Constant  Value=0.3
  Constant6 : Constant  Value=0
  Determine reference vector (U*) : Subsystem
  INFO : Subsystem
      mask Display: disp('?')
  SV Modulator Pattern #1 : Subsystem
  Sector Number : Outport  VectorParamsAs1DForOutWhenUnconnected=off
  Ta Tb T0 normalized : Outport  Port=2  VectorParamsAs1DForOutWhenUnconnected=off
  wires:
  SV Modulator Pattern #1/1(Sector Number) -> Sector Number/1
  SV Modulator Pattern #1/2(Ta Tb T0 normalized) -> Ta Tb T0 normalized/1
  U_angle/1 -> Determine reference vector (U*)/2(In2)
  Determine reference vector (U*)/2(alpha) -> SV Modulator Pattern #1/2(alpha)
  Constant6/1 -> Determine reference vector (U*)/5(Pha_Init)
  Determine reference vector (U*)/1(m) -> SV Modulator Pattern #1/1(m)
  Constant5/1 -> Determine reference vector (U*)/3(m_Int)
  Constant4/1 -> Determine reference vector (U*)/4(Freq_Int)
  U_mag/1 -> Determine reference vector (U*)/1(In1)

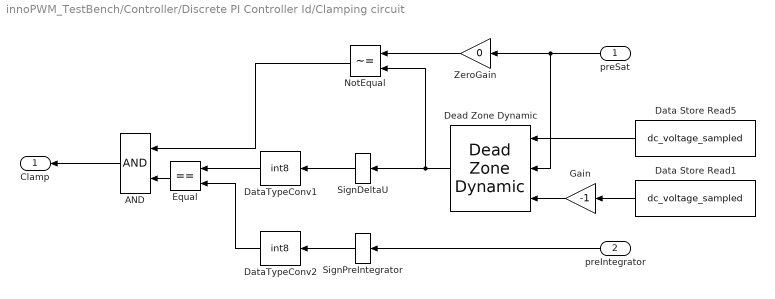
== system innoPWM_TestBench/Controller/Discrete PI Controller Id/Clamping circuit ==
  preSat : Inport  DisableCoverage=on
  preIntegrator : Inport  DisableCoverage=on  Port=2
  AND : Logic  DisableCoverage=on
  Data Store Read1 : DataStoreRead  DataStoreName=dc_voltage_sampled  IndexOptions=Index vector (dialog)  Indices=1  OutputSizes=1
  Data Store Read5 : DataStoreRead  DataStoreName=dc_voltage_sampled  IndexOptions=Index vector (dialog)  Indices=1  OutputSizes=1
  DataTypeConv1 : DataTypeConversion  DisableCoverage=on  OutDataTypeStr=int8  LockScale=on
  DataTypeConv2 : DataTypeConversion  DisableCoverage=on  OutDataTypeStr=int8  SaturateOnIntegerOverflow=off  RndMeth=Floor
  Dead Zone Dynamic : simulink/Discontinuities/Dead Zone Dynamic
      settings: SourceProductBaseCode=SL
  Equal : RelationalOperator  DisableCoverage=on  Operator===
  Gain : Gain  Gain=-1
  NotEqual : RelationalOperator  DisableCoverage=on  Operator=~=
  SignDeltaU : Signum  DisableCoverage=on
  SignPreIntegrator : Signum  DisableCoverage=on
  ZeroGain : Gain  DisableCoverage=on  Gain=0  SaturateOnIntegerOverflow=on  OutDataTypeStr=Inherit: Same as input  ParamDataTypeStr=Inherit: Same as input
  Clamp : Outport  DisableCoverage=on  VectorParamsAs1DForOutWhenUnconnected=off
  wires:
  preSat/1 -> Dead Zone Dynamic/2, ZeroGain/1
  preIntegrator/1 -> SignPreIntegrator/1
  ZeroGain/1 -> NotEqual/1
  Dead Zone Dynamic/1 -> NotEqual/2, SignDeltaU/1
  SignDeltaU/1 -> DataTypeConv1/1
  DataTypeConv1/1 -> Equal/1
  SignPreIntegrator/1 -> DataTypeConv2/1
  DataTypeConv2/1 -> Equal/2
  NotEqual/1 -> AND/1
  Equal/1 -> AND/2
  AND/1 -> Clamp/1
  Data Store Read1/1 -> Gain/1
  Data Store Read5/1 -> Dead Zone Dynamic/1
  Gain/1 -> Dead Zone Dynamic/3

== system innoPWM_TestBench/Controller/Discrete PI Controller Iq/Clamping circuit ==
  preSat : Inport  DisableCoverage=on
  preIntegrator : Inport  DisableCoverage=on  Port=2
  AND : Logic  DisableCoverage=on
  Data Store Read1 : DataStoreRead  DataStoreName=dc_voltage_sampled  IndexOptions=Index vector (dialog)  Indices=1  OutputSizes=1
  Data Store Read5 : DataStoreRead  DataStoreName=dc_voltage_sampled  IndexOptions=Index vector (dialog)  Indices=1  OutputSizes=1
  DataTypeConv1 : DataTypeConversion  DisableCoverage=on  OutDataTypeStr=int8  LockScale=on
  DataTypeConv2 : DataTypeConversion  DisableCoverage=on  OutDataTypeStr=int8  SaturateOnIntegerOverflow=off  RndMeth=Floor
  Dead Zone Dynamic : simulink/Discontinuities/Dead Zone Dynamic
      settings: SourceProductBaseCode=SL
  Equal : RelationalOperator  DisableCoverage=on  Operator===
  Gain : Gain  Gain=-1
  NotEqual : RelationalOperator  DisableCoverage=on  Operator=~=
  SignDeltaU : Signum  DisableCoverage=on
  SignPreIntegrator : Signum  DisableCoverage=on
  ZeroGain : Gain  DisableCoverage=on  Gain=0  SaturateOnIntegerOverflow=on  OutDataTypeStr=Inherit: Same as input  ParamDataTypeStr=Inherit: Same as input
  Clamp : Outport  DisableCoverage=on  VectorParamsAs1DForOutWhenUnconnected=off
  wires:
  Gain/1 -> Dead Zone Dynamic/3
  Data Store Read5/1 -> Dead Zone Dynamic/1
  Data Store Read1/1 -> Gain/1
  AND/1 -> Clamp/1
  Equal/1 -> AND/2
  NotEqual/1 -> AND/1
  DataTypeConv2/1 -> Equal/2
  SignPreIntegrator/1 -> DataTypeConv2/1
  DataTypeConv1/1 -> Equal/1
  SignDeltaU/1 -> DataTypeConv1/1
  Dead Zone Dynamic/1 -> SignDeltaU/1, NotEqual/2
  ZeroGain/1 -> NotEqual/1
  preIntegrator/1 -> SignPreIntegrator/1
  preSat/1 -> ZeroGain/1, Dead Zone Dynamic/2

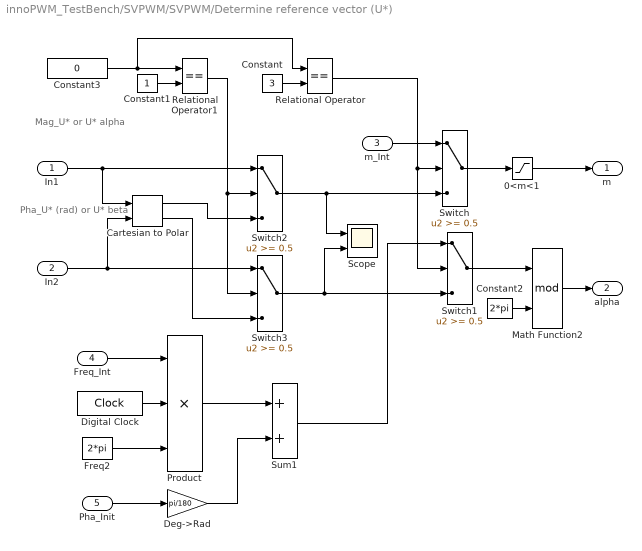
== system innoPWM_TestBench/SVPWM/SVPWM/Determine reference vector (U*) ==
  note: Pha_U* (rad)
      | or
      | U* beta
  note: Mag_U*
      | or
      | U* alpha
  In1 : Inport
  In2 : Inport  Port=2
  m_Int : Inport  Port=3
  Freq_Int : Inport  Port=4
  Pha_Init : Inport  Port=5
  "0<m<1 " : Saturate  UpperLimit=1  LowerLimit=0
  Cartesian to Polar : simulink_extras/Transformations/Cartesian to Polar
  Constant : Constant  Value=3
  Constant1 : Constant
  Constant2 : Constant  Value=2*pi
  Constant3 : Constant  Value=0
  Deg->Rad : Gain  Gain=pi/180  SaturateOnIntegerOverflow=on  OutDataTypeStr=Inherit: Same as input  ParamDataTypeStr=Inherit: Same as input
  Digital Clock : DigitalClock  SampleTime=-1
  Freq2 : Constant  Value=2*pi
  Math Function2 : Math  Operator=mod  SignedPower=on
  Product : Product  Inputs=***  InputSameDT=on  SaturateOnIntegerOverflow=on  OutDataTypeStr=Inherit: Same as first input
  Relational Operator : RelationalOperator  Operator===  InputSameDT=off
  Relational Operator1 : RelationalOperator  Operator===  InputSameDT=off
  Scope : Scope  NumInputPorts=2
  Sum1 : Sum  InputSameDT=on  SaturateOnIntegerOverflow=on  OutDataTypeStr=Inherit: Same as first input
  Switch{,1..3} (4 alike) : Switch  Threshold=0.5  InputSameDT=off
  m : Outport  VectorParamsAs1DForOutWhenUnconnected=off
  alpha : Outport  Port=2  VectorParamsAs1DForOutWhenUnconnected=off
  wires:
  Digital Clock/1 -> Product/2
  Switch1/1 -> Math Function2/1
  Sum1/1 -> Switch1/1
  Math Function2/1 -> alpha/1
  Constant2/1 -> Math Function2/2
  Relational Operator1/1 -> Switch3/2, Switch2/2
  Cartesian to Polar/2 -> Switch3/3
  Cartesian to Polar/1 -> Switch2/3
  Switch2/1 -> Scope/1, Switch/3
  Constant3/1 -> Relational Operator/1, Relational Operator1/1
  Constant1/1 -> Relational Operator1/2
  Relational Operator/1 -> Switch/2, Switch1/2
  Constant/1 -> Relational Operator/2
  m_Int/1 -> Switch/1
  In2/1 -> Switch3/1, Cartesian to Polar/2
  In1/1 -> Switch2/1, Cartesian to Polar/1
  "0<m<1 "/1 -> m/1
  Switch/1 -> "0<m<1 "/1
  Freq2/1 -> Product/3
  Freq_Int/1 -> Product/1
  Deg->Rad/1 -> Sum1/2
  Pha_Init/1 -> Deg->Rad/1
  Product/1 -> Sum1/1
  Switch3/1 -> Scope/2, Switch1/3

== system innoPWM_TestBench/SVPWM/SVPWM/INFO ==
  note: Pattern #2:
      | With this pattern, identified as "Hardware-Determined" by Texas Instruments, there is always one PWM channel staying constant for the entire PWM period.
      |  So the number of switching times for this pattern is less than pattern #1. As a result, switching losses will be reduced with Pattern #2.
  note: Pattern #1:
      | With this pattern, identified as "Software-Determined" by Texas Instruments, each PWM channel switches twice per every PWM period.
  note: --------------------------------------------------------------------------------------------------------------------------------------------------------------------
  note: Reference: Application Report SPRA524
      | Space-Vector PWM with TMS320C24x Using H/W & S/W Determined Switching Patterns
      | Zhenyu Yu, Texas Instruments
  note: The objective of the SV PWM technique is to approximate the reference voltage vector (U*) instantaneously
      | by combination of the switching states corresponding to the basic space vectors.
  note: U7 = 1 1 1
  note: Q1 Q3 Q5
  note: --------------------------------------------------------
  note: Three-Phase VSC Diagram
  note: -
  note: +
  note: --------------------------------------------------------
  note: |
      | |
      | |
  note: ---Vc
  note: |
      | |
      | |
  note: |
      | |
      | |
      | |
      | |
      | |
  note: [Q6]
  note: [Q5]
  note: |
      | |
      | |
  note: ---Vb
  note: |
      | |
      | |
  note: |
      | |
      | |
      | |
      | |
      | |
  note: [Q4]
  note: [Q3]
  note: |
      | |
      | |
  note: ---Va
  note: |
      | |
      | |
  note: |
      | |
      | |
      | |
      | |
      | |
  note: [Q2]
  note: [Q1]
  note: Vdc
  note: [n] = Sector number
  note: [2]
  note: Basic Space Vectors and Switching States
  note: U4 = 0 1 1
  note: U5 = 0 0 1
  note: U6 = 1 0 1
  note: U0 = 0 0 0
  note: U3 = 0 1 0
  note: U2 = 1 1 0
  note: U1 = 1 0 0
  note: [6]
  note: [5]
  note: [4]
  note: [3]
  note: [1]
  note: 3                       2
      |       3                   2
      |         3               2
      |           3           2
      |             3       2
      |               3   2
      | 4 4 4 4 4 4 4 4 0 1 1 1 1 1 1 1 1
      |               5   6
      |             5       6
      |           5           6
      |         5               6
      |       5                   6
      |     5                       6
  note: Two symmetrical switching patterns have been implemented:

== system innoPWM_TestBench/SVPWM/SVPWM/SV Modulator Pattern #1 ==
  m : Inport
  alpha : Inport  Port=2
  "Compute time duration of switching states (Ta,Tb,To) " : Subsystem
  "Determine the sector of U* based on alpha (rad). Also, determine if the sector number is odd" : Subsystem
  INFO : Subsystem
      mask Display: disp('?')
  Sector Number : Outport  VectorParamsAs1DForOutWhenUnconnected=off
  Ta Tb T0 normalized : Outport  Port=2  VectorParamsAs1DForOutWhenUnconnected=off
  wires:
  m/1 -> "Compute time duration of switching states (Ta,Tb,To) "/2(m)
  alpha/1 -> "Compute time duration of switching states (Ta,Tb,To) "/1(alpha), "Determine the sector of U* based on alpha (rad). Also, determine if the sector number is odd"/1(alpha)
  "Compute time duration of switching states (Ta,Tb,To) "/1(Ta Tb T0 normalized) -> Ta Tb T0 normalized/1
  "Determine the sector of U* based on alpha (rad). Also, determine if the sector number is odd"/2(Odd_S) -> "Compute time duration of switching states (Ta,Tb,To) "/4(Odd_S)
  "Determine the sector of U* based on alpha (rad). Also, determine if the sector number is odd"/1(Sn) -> Sector Number/1, "Compute time duration of switching states (Ta,Tb,To) "/3(Sn)

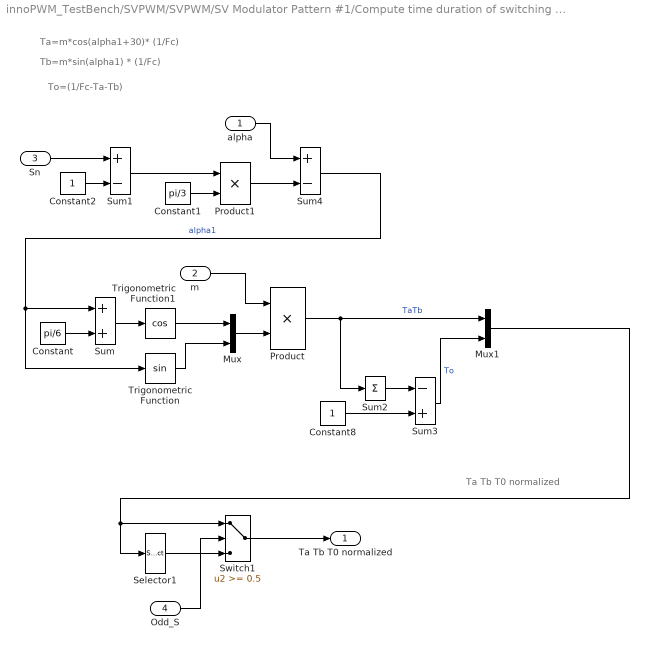
== system innoPWM_TestBench/SVPWM/SVPWM/SV Modulator Pattern #1/Compute time duration of switching states (Ta,Tb,To)  ==
  note: Ta Tb T0 normalized
  note: To=(1/Fc-Ta-Tb)
  note: Tb=m*sin(alpha1) * (1/Fc)
  note: Ta=m*cos(alpha1+30)* (1/Fc)
  alpha : Inport
  m : Inport  Port=2
  Sn : Inport  Port=3
  Odd_S : Inport  Port=4
  Constant : Constant  Value=pi/6
  Constant1 : Constant  Value=pi/3
  Constant2 : Constant
  Constant8 : Constant
  Mux : Mux  Inputs=2
  Mux1 : Mux  Inputs=2
  Product : Product  SaturateOnIntegerOverflow=on  OutDataTypeStr=Inherit: Same as first input
  Product1 : Product  SaturateOnIntegerOverflow=on  OutDataTypeStr=Inherit: Same as first input
  Selector1 : Selector  InputPortWidth=3  IndexOptions=Index vector (dialog)  Indices=[2 1 3]  OutputSizes=1
  Sum : Sum  SaturateOnIntegerOverflow=on
  Sum1 : Sum  Inputs=+-  SaturateOnIntegerOverflow=on
  Sum2 : Sum  Inputs=1  SaturateOnIntegerOverflow=on
  Sum3 : Sum  Inputs=-+  SaturateOnIntegerOverflow=on
  Sum4 : Sum  Inputs=+-  SaturateOnIntegerOverflow=on
  Switch1 : Switch  Threshold=0.5  InputSameDT=off
  Trigonometric Function : Trigonometry
  Trigonometric Function1 : Trigonometry  Operator=cos
  Ta Tb T0 normalized : Outport  VectorParamsAs1DForOutWhenUnconnected=off
  wires:
  Odd_S/1 -> Switch1/2
  Switch1/1 -> Ta Tb T0 normalized/1
  Selector1/1 -> Switch1/3
  Mux1/1 -> Selector1/1, Switch1/1
  Constant/1 -> Sum/2
  Sum4/1 -> Trigonometric Function/1, Sum/1  "alpha1"
  Sum3/1 -> Mux1/2  "To"
  Product/1 -> Sum2/1, Mux1/1  "TaTb"
  alpha/1 -> Sum4/1
  Product1/1 -> Sum4/2
  Constant2/1 -> Sum1/2
  Sn/1 -> Sum1/1
  Constant1/1 -> Product1/2
  Sum1/1 -> Product1/1
  Constant8/1 -> Sum3/2
  Sum2/1 -> Sum3/1
  Sum/1 -> Trigonometric Function1/1
  m/1 -> Product/1
  Mux/1 -> Product/2
  Trigonometric Function/1 -> Mux/2
  Trigonometric Function1/1 -> Mux/1

== system innoPWM_TestBench/SVPWM/SVPWM/SV Modulator Pattern #1/Determine the sector of U* based on alpha (rad). Also, determine if the sector number is odd ==
  alpha : Inport
  Constant1 : Constant  Value=2
  Look-Up Table : Lookup  InputValues=[0:pi/3:5*pi/3]  Table=[1:6]  LookUpMeth=Interpolation-Use End Values
  Math Function1 : Math  Operator=mod  SignedPower=on
  Rounding Function : Rounding
  Sn : Outport  VectorParamsAs1DForOutWhenUnconnected=off
  Odd_S : Outport  Port=2  VectorParamsAs1DForOutWhenUnconnected=off
  wires:
  alpha/1 -> Look-Up Table/1
  Math Function1/1 -> Odd_S/1
  Constant1/1 -> Math Function1/2
  Rounding Function/1 -> Sn/1, Math Function1/1
  Look-Up Table/1 -> Rounding Function/1

== system innoPWM_TestBench/SVPWM/SVPWM/SV Modulator Pattern #1/INFO ==
  note: Interval 7
  note: Interval 6
  note: Interval 5
  note: Interval 4
  note: Interval 3
  note: Interval 2
  note: Interval 1
  note: zero
      | space vector
      | (Q1 Q3 Q5 =0)
  note: 1st basic
      | space vector
  note: 2nd basic
      | space vector
  note: zero
      | space vector
      | (Q1 Q3 Q5 =1)
  note: zero
      | space vector
      | (Q1 Q3 Q5 =0)
  note: 2nd basic
      | space vector
  note: 1st basic
      | space vector
  note: Pattern #1 implements the following symmetrical switching pattern:
      | total duration = 1 PWM period (Tpwm = 1/Fc)
  note: |
      | |
      | |
      | |
      | |
      | |
      | |
      | |
      | |
      | |
  note: |
      | |
      | |
      | |
      | |
      | |
      | |
      | |
      | |
      | |
  note: |
      | |
      | |
      | |
      | |
      | |
      | |
      | |
      | |
      | |
  note: |
      | |
      | |
      | |
      | |
      | |
      | |
      | |
      | |
      | |
  note: |
      | |
      | |
      | |
      | |
      | |
      | |
      | |
      | |
      | |
  note: |
      | |
      | |
      | |
      | |
      | |
      | |
      | |
      | |
      | |
  note: Ta/2
  note: To/4
  note: Tb/2
  note: To/2
  note: Tb/2
  note: Ta/2
  note: To/4
  note: Ta=m*cos(alpha+30)* (1/Fc)
  note: Tb=m*sin(alpha) * (1/Fc)
  note: To=(1/Fc-Ta-Tb)
  note: where:
      | Fc = Chopping frequency
      | m = modulation index
      | alpha = angle between reference vector U* and
      | 1st basic space vector

== matlab function innoPWM_TestBench/Controller/Subsystem/MATLAB Function1 ==
  data: fc input; fpwm input; tau output
function tau = fcn(fc, fpwm)

delta_t = 1/fpwm;
tau     = 1/(2*pi*fc);
alpha   = delta_t / (tau+delta_t);
tau     = -(delta_t/(log(alpha)));

end

== matlab function innoPWM_TestBench/Controller/Subsystem/MATLAB Function2 ==
  data: w input; g output; tau input; a output
function [g,a] = fcn(w,tau)
wt = w*tau;
g = wt/(1+wt);
a = 1-2*g;
